simulink library "powerlib_modelsV2"  (Simulink 6.0)
settings: Solver=ode45  SolverMode=SingleTasking  StartTime=0.0  StopTime=10.0  RelTol=1e-3
values from neighbouring files (symbols this model uses):
  Ts = get(handles.edit1,'string')    [powergui.m]
undefined symbols (not defined in the file or in its folder): A, Ac, B, Bc, C, Cc, Cs, Current, damp, Dc, Dd, DiscIntNeverNeededParam, dref, dwo, exc, F, fb, gate, GH, GHd, GI, GId, GL, GLd, H, HT, hyd, ib, ib2, io, isfinite, j, K, Kd, Kg, L, Lad, Laq, lim, LIM, Ll, Llfd, Llkd, Llkq1, Llkq2, Llr, Lls, LowerFlux, N, N2, Nb, Nb2, nb_arm, p, Par_HarmoA_pu, Par_HarmoB_pu, Par_Timing_Harmo, Par_Timing_Variation, Par_Vps, Pb ... (+57)
libraries: powerlib_extras x14
(part 7 of 11)

== system powerlib_modelsV2/Continuous/simplified_sync_mach/Subsystem ==
  i : Inport  Port=1  LatchInput=off
  v : Inport  Port=2  LatchInput=off
  e : Inport  Port=3  LatchInput=off
  theta : Inport  Port=4  LatchInput=off
  wm : Inport  Port=5  LatchInput=off
  Pe : Inport  Port=6  LatchInput=off
  Gain : Gain  Gain=[ ib2*ones(3,1); Vb3*ones(6,1); 1; Nb; Pb ]  SaturateOnIntegerOverflow=on
  Mux : Mux  Inputs=[ 3 3 3 1 1 1 ]
  * : Outport  InitialOutput=0
  wires:
  Gain/1 -> */1
  Mux/1 -> Gain/1
  Pe/1 -> Mux/6
  wm/1 -> Mux/5
  theta/1 -> Mux/4
  e/1 -> Mux/3
  v/1 -> Mux/2
  i/1 -> Mux/1

== system powerlib_modelsV2/Continuous/simplified_sync_mach/Vt ==
  note: This subsystem either converts 2 line-to-line voltages to 3 line-to-neutral voltages (internal neutral)
      | and computes floating neutral voltage or directly passes Van,Vbn,Vcn if 4-wire connection.
  V : Inport  Port=1  LatchInput=off
  1_Vb : Gain  Gain=1/Vb  SaturateOnIntegerOverflow=on
  Constant : Constant  Orientation=left  Value=v6==1
  Constant1 : Constant  Value=0
  Constant2 : Constant  Value=0
  Data Type  Conversion1 : DataTypeConversion  Orientation=left  SaturateOnIntegerOverflow=on  RndMeth=Zero
  Data Type  Conversion2 : DataTypeConversion  SaturateOnIntegerOverflow=on  RndMeth=Zero
  Fcn : Fcn  Expr=u[1]
  Fcn1 : Fcn  Expr=u[2]
  Fcn2 : Fcn  Expr=u[3]
  Gain : Gain  Gain=1/3  SaturateOnIntegerOverflow=on
  LL2LN : Subsystem  TreatAsAtomicUnit=on
  Logical Operator : Logic  Operator=NOT
  Mux : Mux  Inputs=2
  Mux1 : Mux  Inputs=3
  Product : Product  SaturateOnIntegerOverflow=on  InputSameDT=on
  Sum : Sum  Inputs=+  SaturateOnIntegerOverflow=on  InputSameDT=on
  Sum1 : Sum  Inputs=|++  SaturateOnIntegerOverflow=on  InputSameDT=on
  Switch2 : Switch  Threshold=0.5  InputSameDT=on
  Vn : Outport  InitialOutput=0
  Vabc : Outport  Port=2  InitialOutput=0
  wires:
  Data Type  Conversion2/1 -> Product/1
  Logical Operator/1 -> Data Type  Conversion2/1
  Data Type  Conversion1/1 -> Logical Operator/1
  Constant/1 -> Data Type  Conversion1/1, LL2LN/Enable, Switch2/2
  Sum/1 -> Gain/1
  Gain/1 -> Switch2/1
  Constant2/1 -> Switch2/3
  Switch2/1 -> Vn/1
  LL2LN/1(Out1) -> Sum/1, Sum1/1
  Sum1/1 -> Vabc/1
  Constant1/1 -> Mux/2
  Mux/1 -> Fcn/1, Fcn1/1, Fcn2/1
  Fcn/1 -> Mux1/1
  Fcn1/1 -> Mux1/2
  Fcn2/1 -> Mux1/3
  Mux1/1 -> Product/2
  Product/1 -> Sum1/2
  V/1 -> 1_Vb/1
  1_Vb/1 -> LL2LN/1(In1), Mux/1

== system powerlib_modelsV2/Continuous/simplified_sync_mach/Z ==
  note: This subsystem models the internal impedance of
      | the machine, which consists of  a series RL circuit.
  e : Inport  Port=1  LatchInput=off
  v : Inport  Port=2  LatchInput=off
  1/L : Gain  Gain=web_psb/L  SaturateOnIntegerOverflow=on
  Integrator3 : Integrator  InitialCondition=io
  R : Gain  Orientation=left  Gain=R  SaturateOnIntegerOverflow=on
  Sum5 : Sum  Inputs=-+-  SaturateOnIntegerOverflow=on  InputSameDT=on
  i : Outport  InitialOutput=0
  wires:
  Integrator3/1 -> i/1, R/1
  1/L/1 -> Integrator3/1
  v/1 -> Sum5/3
  Sum5/1 -> 1/L/1
  R/1 -> Sum5/1
  e/1 -> Sum5/2

== system powerlib_modelsV2/Continuous/simplified_sync_mach/gen ==
  note: This subsystem generates the 3 line-to-neutral voltages inside the machine.
  theta : Inport  Port=1  LatchInput=off
  E : Inport  Port=2  LatchInput=off
  Vn : Inport  Port=3  LatchInput=off
  1_Vb2 : Gain  Gain=1/Vb2  SaturateOnIntegerOverflow=on
  Mux : Mux  Inputs=3
  Product : Product  SaturateOnIntegerOverflow=on  InputSameDT=on
  Sum : Sum  Inputs=|++  SaturateOnIntegerOverflow=on  InputSameDT=on
  Sum1 : Sum  Orientation=down  Inputs=--  SaturateOnIntegerOverflow=on  InputSameDT=on
  rem(wt,2pi) : Fcn  Expr=rem(u[1],2*pi)
  sin(a) : Fcn  Expr=sin(u)
  sin(b) : Fcn  Expr=sin(u-pi23)
  e : Outport  InitialOutput=0
  wires:
  rem(wt,2pi)/1 -> sin(a)/1, sin(b)/1
  theta/1 -> rem(wt,2pi)/1
  sin(a)/1 -> Sum1/2, Mux/1
  Sum1/1 -> Mux/3
  sin(b)/1 -> Sum1/1, Mux/2
  E/1 -> 1_Vb2/1
  1_Vb2/1 -> Product/2
  Vn/1 -> Sum/2
  Mux/1 -> Product/1
  Product/1 -> Sum/1
  Sum/1 -> e/1

== system powerlib_modelsV2/Continuous/simplified_sync_mach/mechanics ==
  Pm : Inport  Port=1  LatchInput=off
  Pe : Inport  Port=2  LatchInput=off
  1_(2*H) : Gain  Gain=1/(2*H)  SaturateOnIntegerOverflow=on
  1_Pb : Gain  Gain=1/Pb  SaturateOnIntegerOverflow=on
  Gain : Gain  Orientation=left  Gain=Kd  SaturateOnIntegerOverflow=on
  Integrator : Integrator  InitialCondition=dwo
  Integrator1 : Integrator  InitialCondition=tho
  Mux1 : Mux  Inputs=2
  Sum : Sum  SaturateOnIntegerOverflow=on  InputSameDT=on
  Sum1 : Sum  Inputs=+-  SaturateOnIntegerOverflow=on  InputSameDT=on
  Sum2 : Sum  Inputs=-+  SaturateOnIntegerOverflow=on  InputSameDT=on
  div : Fcn  Expr=u[2]/u[1]
      mask Display: disp('division')
  nom. speed : Constant
  web_psb : Gain  Gain=web_psb  SaturateOnIntegerOverflow=on
  theta_e : Outport  InitialOutput=0
  wm : Outport  Port=2  InitialOutput=0
  wires:
  Pm/1 -> 1_Pb/1
  1_Pb/1 -> Sum2/2
  web_psb/1 -> Integrator1/1
  Integrator1/1 -> theta_e/1
  Mux1/1 -> div/1
  Pe/1 -> Sum2/1
  Sum2/1 -> Mux1/2
  Sum/1 -> Mux1/1, wm/1, web_psb/1
  1_(2*H)/1 -> Integrator/1
  div/1 -> Sum1/1
  Gain/1 -> Sum1/2
  Sum1/1 -> 1_(2*H)/1
  Integrator/1 -> Sum/2, Gain/1
  nom. speed/1 -> Sum/1

== system powerlib_modelsV2/Continuous/simplified_sync_mach/wattmeter ==
  note: This subsystem computes the total electrical
      | power delivered or absorbed by the machine.
  i : Inport  Port=1  LatchInput=off
  v : Inport  Port=2  LatchInput=off
  2_3 : Gain  Gain=2/3  SaturateOnIntegerOverflow=on
  Product : Product  SaturateOnIntegerOverflow=on  InputSameDT=on
  Sum : Sum  Inputs=+  SaturateOnIntegerOverflow=on  InputSameDT=on
  Pe : Outport  InitialOutput=0
  wires:
  Product/1 -> Sum/1
  i/1 -> Product/1
  v/1 -> Product/2
  Sum/1 -> 2_3/1
  2_3/1 -> Pe/1

== system powerlib_modelsV2/Continuous/synchronous_machine/Delta angle ==
  Vq : Inport  Port=1  PortDimensions=1  LatchInput=off
  Vd : Inport  Port=2  PortDimensions=1  LatchInput=off
  Cartesian to Polar : Subsystem
      mask Type: Cart2Polar
      mask Description:
      | Transformation from cartesian to polar coordinates.
      | [x, y] -> [r, theta]
      | 
      | r = sqrt(x^2 + y^2);
      | theta = atan(y/x);
      mask Help: Unmask this block for more help.
      mask Display: plot(0,0,100,100,[24,20,15,20,20],[85,95,85,95,20],[80,20,95,85,95,85],[70,20,20,15,20,24],[56,56,55,52,50,46],[20,26,31,35,38,42])
  Radians to Degrees : Subsystem
      mask Type: RadiansToDegrees
      mask Description:
      | Conversion from Radians to Degrees.
      | 
      | D=180/pi*R
      mask Help: This block converts from Radians to Degrees.
      mask Display: disp('R2D')
  Terminator2 : Terminator
  delta : Outport
  wires:
  Cartesian to Polar/2(theta) -> Radians to Degrees/1(Radians in)
  Cartesian to Polar/1(r) -> Terminator2/1
  Vq/1 -> Cartesian to Polar/1(x)
  Radians to Degrees/1(Degrees out) -> delta/1  "delta"
  Vd/1 -> Cartesian to Polar/2(y)

== system powerlib_modelsV2/Continuous/synchronous_machine/PQ ==
  note: PQ Measurement:
  note: Q = Vq*Id-Vd*Iq
  note: P = Vd*Id + Vq*Iq
  Vq : Inport  Port=1  PortDimensions=1  LatchInput=off
  Vd : Inport  Port=2  PortDimensions=1  LatchInput=off
  Iq : Inport  Port=3  PortDimensions=2  LatchInput=off
  Demux1 : Demux  Outputs=[1,1]
  Gain : Gain  Gain=Gain1  SaturateOnIntegerOverflow=on
  Gain1 : Gain  Gain=Gain1  SaturateOnIntegerOverflow=on
  Product{2..5} (4 alike) : Product  SaturateOnIntegerOverflow=on  InputSameDT=on
  Sum : Sum  SaturateOnIntegerOverflow=on  InputSameDT=on
  Sum1 : Sum  Inputs=+-  SaturateOnIntegerOverflow=on  InputSameDT=on
  Peo : Outport
  Qeo : Outport  Port=2
  wires:
  Demux1/2 -> Product4/2, Product3/2
  Vq/1 -> Product4/1, Product2/1
  Vd/1 -> Product5/1, Product3/1
  Sum1/1 -> Gain1/1  "Qeo"
  Sum/1 -> Gain/1  "Peo"
  Product5/1 -> Sum1/2
  Product4/1 -> Sum1/1
  Product3/1 -> Sum/2
  Product2/1 -> Sum/1
  Gain/1 -> Peo/1
  Gain1/1 -> Qeo/1
  Iq/1 -> Demux1/1
  Demux1/1 -> Product2/2, Product5/2

== system powerlib_modelsV2/Continuous/synchronous_machine/Subsystem ==
  Vf : Inport  Port=1  PortDimensions=1  LatchInput=off
  Constant : Constant  Value=excAxis
  Ground2 : Ground
  Switch : Switch  Threshold=1.5  InputSameDT=on
  Switch1 : Switch  Threshold=1.5  InputSameDT=on
  Vkq1 : Outport
  Vfd : Outport  Port=2
  wires:
  Ground2/1 -> Switch1/1, Switch/3
  Vf/1 -> Switch1/3, Switch/1
  Constant/1 -> Switch/2, Switch1/2
  Switch1/1 -> Vfd/1
  Switch/1 -> Vkq1/1

== system powerlib_modelsV2/Continuous/synchronous_machine/abc2qd ==
  note: This subsystem converts Vab and Vbc to Vd,Vq. The sine and cosine com-
      | puted here are sent to the inverse transformation subsystem qd/abc.
  v : Inport  Port=1  PortDimensions=2  LatchInput=off
  theta : Inport  Port=2  PortDimensions=1  LatchInput=off
  1_Vb : Gain  Gain=1/Vb  SaturateOnIntegerOverflow=on
  Elementary Math : ElementaryMath
  Elementary Math1 : ElementaryMath  Operator=cos
  Fcn2 : Fcn  Expr=(u[4]*(2*u[1]+u[2]) + (sqrt3*u[2]*u[3])) * one_third
  Fcn3 : Fcn  Expr=(u[3]*(2*u[1]+u[2]) + (-sqrt3*u[2]*u[4])) * one_third
  Mux1 : Mux  Inputs=[ 2 2 ]
  Mux3 : Mux  Inputs=2
  cos,sin : Outport  InitialOutput=0
  vq : Outport  Port=2  InitialOutput=0
  vd : Outport  Port=3  InitialOutput=0
  wires:
  1_Vb/1 -> Mux1/1
  v/1 -> 1_Vb/1
  Mux1/1 -> Fcn2/1, Fcn3/1
  Mux3/1 -> Mux1/2, cos,sin/1
  theta/1 -> Elementary Math/1, Elementary Math1/1
  Elementary Math/1 -> Mux3/1
  Elementary Math1/1 -> Mux3/2
  Fcn2/1 -> vq/1  "vq"
  Fcn3/1 -> vd/1  "vd"

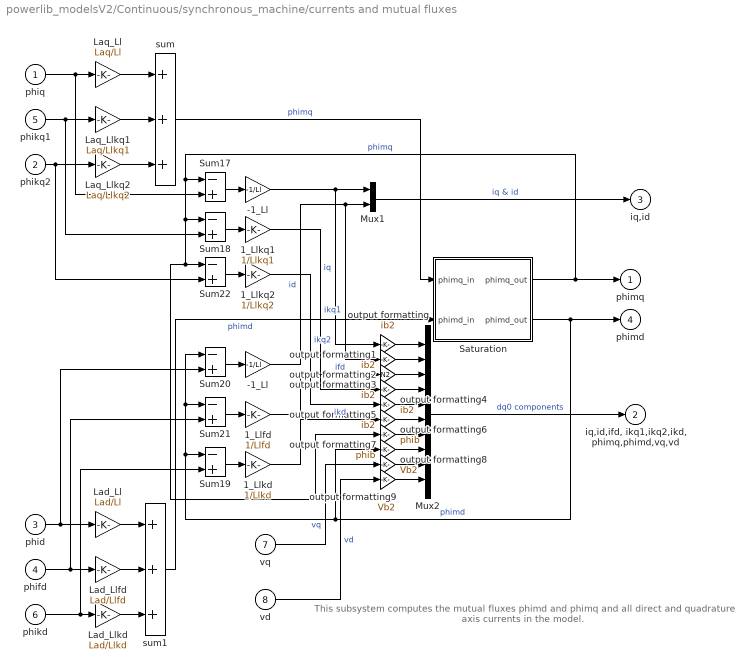
== system powerlib_modelsV2/Continuous/synchronous_machine/currents and mutual fluxes ==
  note: This subsystem computes the mutual fluxes phimd
      | and phimq and all direct and quadrature axis
      | currents in the model.
  phiq : Inport  Port=1  PortDimensions=1  LatchInput=off
  phikq2 : Inport  Port=2  PortDimensions=1  LatchInput=off
  phid : Inport  Port=3  PortDimensions=1  LatchInput=off
  phifd : Inport  Port=4  PortDimensions=1  LatchInput=off
  phikq1 : Inport  Port=5  PortDimensions=1  LatchInput=off
  phikd : Inport  Port=6  PortDimensions=1  LatchInput=off
  vq : Inport  Port=7  PortDimensions=1  LatchInput=off
  vd : Inport  Port=8  PortDimensions=1  LatchInput=off
  -1_Ll : Gain  Gain=-1/Ll  SaturateOnIntegerOverflow=on
  "-1_Ll " : Gain  Gain=-1/Ll  SaturateOnIntegerOverflow=on
  1_Llfd : Gain  Gain=1/Llfd  SaturateOnIntegerOverflow=on
  1_Llkd : Gain  Gain=1/Llkd  SaturateOnIntegerOverflow=on
  1_Llkq1 : Gain  Gain=1/Llkq1  SaturateOnIntegerOverflow=on
  1_Llkq2 : Gain  Gain=1/Llkq2  SaturateOnIntegerOverflow=on
  Lad_Ll : Gain  Gain=Lad/Ll  SaturateOnIntegerOverflow=on
  Lad_Llfd : Gain  Gain=Lad/Llfd  SaturateOnIntegerOverflow=on
  Lad_Llkd : Gain  Gain=Lad/Llkd  SaturateOnIntegerOverflow=on
  Laq_Ll : Gain  Gain=Laq/Ll  SaturateOnIntegerOverflow=on
  Laq_Llkq1 : Gain  Gain=Laq/Llkq1  SaturateOnIntegerOverflow=on
  Laq_Llkq2 : Gain  Gain=Laq/Llkq2  SaturateOnIntegerOverflow=on
  Mux1 : Mux  Inputs=2
  Mux2 : Mux  Inputs=[1,1,1,1,1,1,1,1,1,1]
  Saturation : Subsystem
  Sum{17..22} (6 alike) : Sum  Inputs=-+  SaturateOnIntegerOverflow=on  InputSameDT=on
  output formatting{,1,3..5} (5 alike) : Gain  Gain=ib2  SaturateOnIntegerOverflow=on
  output formatting2 : Gain  Gain=N2  SaturateOnIntegerOverflow=on
  output formatting6 : Gain  Gain=phib  SaturateOnIntegerOverflow=on
  output formatting7 : Gain  Gain=phib  SaturateOnIntegerOverflow=on
  output formatting8 : Gain  Gain=Vb2  SaturateOnIntegerOverflow=on
  output formatting9 : Gain  Gain=Vb2  SaturateOnIntegerOverflow=on
  sum : Sum  Inputs=+++  SaturateOnIntegerOverflow=on  InputSameDT=on
  sum1 : Sum  Inputs=+++  SaturateOnIntegerOverflow=on  InputSameDT=on
  phimq : Outport  InitialOutput=0
  "iq,id,ifd, ikq1,ikq2,ikd, phimq,phimd,vq,vd" : Outport  Port=2  InitialOutput=0
  iq,id : Outport  Port=3  InitialOutput=0
  phimd : Outport  Port=4  InitialOutput=0
  wires:
  Saturation/2(phimd_out) -> Sum19/1, Sum21/1, Sum20/1, output formatting7/1, phimd/1  "phimd"
  Saturation/1(phimq_out) -> Sum17/1, Sum22/1, output formatting6/1, Sum18/1, phimq/1  "phimq"
  sum1/1 -> Saturation/2(phimd_in)  "phimd"
  sum/1 -> Saturation/1(phimq_in)  "phimq"
  1_Llkq2/1 -> output formatting4/1  "ikq2"
  1_Llkq1/1 -> output formatting3/1  "ikq1"
  Sum20/1 -> "-1_Ll "/1
  "-1_Ll "/1 -> Mux1/2, output formatting1/1  "id"
  Sum21/1 -> 1_Llfd/1
  Sum19/1 -> 1_Llkd/1
  1_Llfd/1 -> output formatting2/1  "ifd"
  1_Llkd/1 -> output formatting5/1  "ikd"
  Sum18/1 -> 1_Llkq1/1
  Sum17/1 -> -1_Ll/1
  Sum22/1 -> 1_Llkq2/1
  -1_Ll/1 -> Mux1/1, output formatting/1  "iq"
  Mux1/1 -> iq,id/1  "iq & id"
  Lad_Llkd/1 -> sum1/3
  Lad_Llfd/1 -> sum1/2
  Lad_Ll/1 -> sum1/1
  phifd/1 -> Lad_Llfd/1, Sum21/2
  phid/1 -> Sum20/2, Lad_Ll/1
  phikd/1 -> Lad_Llkd/1, Sum19/2
  phiq/1 -> Laq_Ll/1, Sum17/2
  Laq_Ll/1 -> sum/1
  Laq_Llkq2/1 -> sum/3
  Laq_Llkq1/1 -> sum/2
  phikq2/1 -> Laq_Llkq2/1, Sum22/2
  phikq1/1 -> Laq_Llkq1/1, Sum18/2
  vq/1 -> output formatting8/1  "vq"
  vd/1 -> output formatting9/1  "vd"
  Mux2/1 -> "iq,id,ifd, ikq1,ikq2,ikd, phimq,phimd,vq,vd"/1  "dq0 components"
  output formatting/1 -> Mux2/1
  output formatting1/1 -> Mux2/2
  output formatting2/1 -> Mux2/3
  output formatting3/1 -> Mux2/4
  output formatting4/1 -> Mux2/5
  output formatting5/1 -> Mux2/6
  output formatting6/1 -> Mux2/7
  output formatting7/1 -> Mux2/8
  output formatting8/1 -> Mux2/9
  output formatting9/1 -> Mux2/10

== system powerlib_modelsV2/Continuous/synchronous_machine/mec ==
  note: This subsystem models the mechanical part of the machine.
  note: Attention: Te tjrs en p.u
  "iq,id " : Inport  Port=1  PortDimensions=2  LatchInput=off
  phid : Inport  Port=2  PortDimensions=1  LatchInput=off
  phiq : Inport  Port=3  PortDimensions=1  LatchInput=off
  Pm : Inport  Port=4  PortDimensions=1  LatchInput=off
  1_(2H) : Gain  Gain=1/(2*H)  SaturateOnIntegerOverflow=on
  1_Pb : Gain  Gain=1/Pb  SaturateOnIntegerOverflow=on
  Clock : Clock
      settings: Decimation=10
  F : Gain  Orientation=left  Gain=F  SaturateOnIntegerOverflow=on
  Fcn1 : Fcn  Expr=rem(u,2*pi)
  Integrator : Integrator  InitialCondition=dwo
  Integrator1 : Integrator  InitialCondition=tho
  Integrator2 : Integrator  InitialCondition=tho
  Mux : Mux  Inputs=[ 1 1 2 ]
  Mux1 : Mux  Inputs=2
  Mux2 : Mux  Inputs=[1,1,1,1,1,1]
  Product : Product  SaturateOnIntegerOverflow=on  InputSameDT=on
  Sum : Sum  SaturateOnIntegerOverflow=on  InputSameDT=on
  Sum2 : Sum  Inputs=+--  SaturateOnIntegerOverflow=on  InputSameDT=on
  Sum3 : Sum  SaturateOnIntegerOverflow=on  InputSameDT=on
  Te : Fcn  Expr=u[1]*u[3]-u[2]*u[4]
  div : Fcn  Expr=u[2]/u[1]
      mask Display: disp('/')
  nom. speed : Constant
  theta : Gain  Gain=180/pi  SaturateOnIntegerOverflow=on
  units : Gain  Gain=Nb  SaturateOnIntegerOverflow=on
  units1 : Gain  Gain=Pb  SaturateOnIntegerOverflow=on
  units2 : Gain  Gain=Pb/Nb  SaturateOnIntegerOverflow=on
  web1 : Gain  Gain=web_psb  SaturateOnIntegerOverflow=on
  web2 : Gain  Gain=web_psb  SaturateOnIntegerOverflow=on
  web3 : Gain  Gain=web_psb  SaturateOnIntegerOverflow=on
  misc : Outport  InitialOutput=0
  thetae : Outport  Port=2  InitialOutput=0
  we : Outport  Port=3  InitialOutput=0
  wires:
  Integrator2/1 -> Sum3/1, Mux2/1  "d_theta (rad)"
  web2/1 -> Sum3/2
  Clock/1 -> web2/1
  web1/1 -> Integrator2/1
  Integrator/1 -> web1/1, F/1, Mux2/4, Sum/2  "dw"
  Product/1 -> units1/1  "Pe"
  nom. speed/1 -> Sum/1
  1_(2H)/1 -> Integrator/1
  div/1 -> Sum2/1
  phiq/1 -> Mux/2
  phid/1 -> Mux/1
  "iq,id "/1 -> Mux/3
  Te/1 -> Sum2/2, Product/2, units2/1  "Te"
  Mux/1 -> Te/1
  Mux1/1 -> div/1
  Pm/1 -> 1_Pb/1
  1_Pb/1 -> Mux1/2
  F/1 -> Sum2/3
  Sum2/1 -> 1_(2H)/1
  Sum/1 -> Product/1, web3/1, units/1, we/1, Mux1/1  "n"
  Sum3/1 -> thetae/1
  web3/1 -> Integrator1/1
  Integrator1/1 -> Fcn1/1  "d_theta (rad)"
  Fcn1/1 -> theta/1
  theta/1 -> Mux2/5  "theta"
  Mux2/1 -> misc/1  "Mechanical"
  units/1 -> Mux2/2  "n"
  units1/1 -> Mux2/3  "Pe"
  units2/1 -> Mux2/6  "Te"

== system powerlib_modelsV2/Continuous/synchronous_machine/phid ==
  note: This subsystem computes the direct axis flux phid.
  w : Inport  Port=1  PortDimensions=1  LatchInput=off
  phiq : Inport  Port=2  PortDimensions=1  LatchInput=off
  vd : Inport  Port=3  PortDimensions=1  LatchInput=off
  phimd : Inport  Port=4  PortDimensions=1  LatchInput=off
  Product1 : Product  SaturateOnIntegerOverflow=on  InputSameDT=on
  Rs_Ll : Gain  Gain=Rs/Ll  SaturateOnIntegerOverflow=on
  Sum2 : Sum  Inputs=+++  SaturateOnIntegerOverflow=on  InputSameDT=on
  Sum9 : Sum  Inputs=+-  SaturateOnIntegerOverflow=on  InputSameDT=on
  int : Integrator  InitialCondition=phido
  web_psb : Gain  Gain=web_psb  SaturateOnIntegerOverflow=on
  phid : Outport  InitialOutput=0
  wires:
  phimd/1 -> Sum9/1
  vd/1 -> Sum2/2
  phiq/1 -> Product1/2
  w/1 -> Product1/1
  Product1/1 -> Sum2/1
  Sum9/1 -> Rs_Ll/1
  Rs_Ll/1 -> Sum2/3
  Sum2/1 -> web_psb/1
  web_psb/1 -> int/1
  int/1 -> phid/1, Sum9/2

== system powerlib_modelsV2/Continuous/synchronous_machine/phifd ==
  note: This subsystem computes the field flux phifd.
  vfd : Inport  Port=1  PortDimensions=1  LatchInput=off
  phimd : Inport  Port=2  PortDimensions=1  LatchInput=off
  N : Gain  Gain=N  SaturateOnIntegerOverflow=on
  Rf_Llfd : Gain  Gain=Rf/Llfd  SaturateOnIntegerOverflow=on
  Sum10 : Sum  Inputs=+-  SaturateOnIntegerOverflow=on  InputSameDT=on
  Sum3 : Sum  SaturateOnIntegerOverflow=on  InputSameDT=on
  int : Integrator  InitialCondition=phifdo
  web_psb : Gain  Gain=web_psb  SaturateOnIntegerOverflow=on
  phifd : Outport  InitialOutput=0
  wires:
  N/1 -> Sum3/1
  vfd/1 -> N/1
  Rf_Llfd/1 -> Sum3/2
  Sum10/1 -> Rf_Llfd/1
  phimd/1 -> Sum10/1
  web_psb/1 -> int/1
  int/1 -> phifd/1, Sum10/2
  Sum3/1 -> web_psb/1

== system powerlib_modelsV2/Continuous/synchronous_machine/phikd ==
  note: This subsystem computes the direct axis damper flux phikd.
  phimd : Inport  Port=1  PortDimensions=1  LatchInput=off
  vkd : Inport  Port=2  PortDimensions=1  LatchInput=off
  Rkd_Llkd : Gain  Gain=Rkd/Llkd  SaturateOnIntegerOverflow=on
  Sum11 : Sum  Inputs=-+  SaturateOnIntegerOverflow=on  InputSameDT=on
  Sum4 : Sum  SaturateOnIntegerOverflow=on  InputSameDT=on
  int : Integrator  InitialCondition=phikdo
  web_psb : Gain  Gain=web_psb  SaturateOnIntegerOverflow=on
  phikd : Outport  InitialOutput=0
  wires:
  Rkd_Llkd/1 -> Sum4/1
  Sum11/1 -> Rkd_Llkd/1
  phimd/1 -> Sum11/2
  vkd/1 -> Sum4/2
  web_psb/1 -> int/1
  int/1 -> phikd/1, Sum11/1
  Sum4/1 -> web_psb/1

== system powerlib_modelsV2/Continuous/synchronous_machine/phikq1 ==
  note: This subsystem computes the quadrature axis damper flux phikq.
  phimq : Inport  Port=1  PortDimensions=1  LatchInput=off
  vkq1 : Inport  Port=2  PortDimensions=1  LatchInput=off
  Rkq1_Llkq1 : Gain  Gain=Rkq1/Llkq1  SaturateOnIntegerOverflow=on
  Sum1 : Sum  SaturateOnIntegerOverflow=on  InputSameDT=on
  Sum7 : Sum  Inputs=-+  SaturateOnIntegerOverflow=on  InputSameDT=on
  int : Integrator  InitialCondition=phikq1o
  web_psb : Gain  Gain=web_psb  SaturateOnIntegerOverflow=on
  phikq1 : Outport  InitialOutput=0
  wires:
  int/1 -> Sum7/1, phikq1/1
  web_psb/1 -> int/1
  vkq1/1 -> Sum1/2
  phimq/1 -> Sum7/2
  Sum1/1 -> web_psb/1
  Sum7/1 -> Rkq1_Llkq1/1
  Rkq1_Llkq1/1 -> Sum1/1

== system powerlib_modelsV2/Continuous/synchronous_machine/phikq2 ==
  note: This subsystem computes the quadrature axis damper flux phikq2.
  vkq2 : Inport  Port=1  PortDimensions=1  LatchInput=off
  phimq : Inport  Port=2  PortDimensions=1  LatchInput=off
  Enabled integrator : Subsystem  TreatAsAtomicUnit=on
      mask Display: disp('1/s')
  Rkq2_Llkq2 : Gain  Gain=Rkq2/Llkq2  SaturateOnIntegerOverflow=on
  Sum1 : Sum  SaturateOnIntegerOverflow=on  InputSameDT=on
  Sum7 : Sum  Inputs=-+  SaturateOnIntegerOverflow=on  InputSameDT=on
  web_psb : Gain  Gain=web_psb  SaturateOnIntegerOverflow=on
  wref : Constant  Value=isfinite(Llkq2)
  phikq2 : Outport  InitialOutput=0
  wires:
  wref/1 -> Enabled integrator/Enable
  Enabled integrator/1(Out1) -> phikq2/1, Sum7/1
  web_psb/1 -> Enabled integrator/1(In1)
  Sum7/1 -> Rkq2_Llkq2/1
  vkq2/1 -> Sum1/2
  Rkq2_Llkq2/1 -> Sum1/1
  Sum1/1 -> web_psb/1
  phimq/1 -> Sum7/2

== system powerlib_modelsV2/Continuous/synchronous_machine/phiq ==
  note: This subsystem computes the quadrature axis flux phiq.
  vq : Inport  Port=1  PortDimensions=1  LatchInput=off
  w : Inport  Port=2  PortDimensions=1  LatchInput=off
  phid : Inport  Port=3  PortDimensions=1  LatchInput=off
  phimq : Inport  Port=4  PortDimensions=1  LatchInput=off
  Product2 : Product  SaturateOnIntegerOverflow=on  InputSameDT=on
  Rs_Ll : Gain  Gain=Rs/Ll  SaturateOnIntegerOverflow=on
  Sum : Sum  Inputs=+-+  SaturateOnIntegerOverflow=on  InputSameDT=on
  Sum6 : Sum  Inputs=+-  SaturateOnIntegerOverflow=on  InputSameDT=on
  int1 : Integrator  InitialCondition=phiqo
  web_psb : Gain  Gain=web_psb  SaturateOnIntegerOverflow=on
  phiq : Outport  InitialOutput=0
  wires:
  Sum/1 -> web_psb/1
  Rs_Ll/1 -> Sum/3
  Sum6/1 -> Rs_Ll/1
  Product2/1 -> Sum/2
  vq/1 -> Sum/1
  w/1 -> Product2/1
  phid/1 -> Product2/2
  phimq/1 -> Sum6/1
  web_psb/1 -> int1/1
  int1/1 -> phiq/1, Sum6/2

== system powerlib_modelsV2/Continuous/synchronous_machine/qd2abc ==
  note: This subsystem converts id,iq to ia,ib,ic.
  sin,cos : Inport  Port=1  PortDimensions=2  LatchInput=off
  iq,id : Inport  Port=2  PortDimensions=2  LatchInput=off
  Fcn : Fcn  Expr=u[3]*u[2] + u[4]*u[1]
  Fcn1 : Fcn  Expr=(u[2]*(-u[3]-sqrt3*u[4]) + u[1]*(sqrt3*u[3]-u[4]))*0.5
  Mux : Mux  Inputs=[ 2 2 ]
  Mux1 : Mux  Inputs=[1,1,1]
  Mux1_ : Mux  Inputs=3
  Sum : Sum  Orientation=down  Inputs=--  SaturateOnIntegerOverflow=on  InputSameDT=on
  ib : Gain  Gain=ib  SaturateOnIntegerOverflow=on
  output formatting : Gain  Gain=ib2  SaturateOnIntegerOverflow=on
  output formatting1 : Gain  Gain=ib2  SaturateOnIntegerOverflow=on
  output formatting2 : Gain  Gain=ib2  SaturateOnIntegerOverflow=on
  is(A) : Outport  InitialOutput=0
  is(pu) : Outport  Port=2  InitialOutput=0
  wires:
  iq,id/1 -> Mux/2
  sin,cos/1 -> Mux/1
  Mux/1 -> Fcn1/1, Fcn/1
  Mux1_/1 -> ib/1
  Sum/1 -> Mux1_/3, output formatting2/1  "is_c"
  Fcn/1 -> Sum/1, Mux1_/1, output formatting/1  "is_a"
  Fcn1/1 -> Sum/2, Mux1_/2, output formatting1/1  "is_b"
  ib/1 -> is(A)/1
  Mux1/1 -> is(pu)/1  "Stator currents"
  output formatting/1 -> Mux1/1  "is_a"
  output formatting1/1 -> Mux1/2  "is_b"
  output formatting2/1 -> Mux1/3  "is_c"

== system powerlib_modelsV2/Continuous/thyristor (logical)/Break Alg. Loop ==
  In1 : Inport  Port=1  LatchInput=off
  0 2 : Constant  Value=0.001
  Data Type  Conversion : DataTypeConversion  SaturateOnIntegerOverflow=on  RndMeth=Zero
  Data Type  Conversion1 : DataTypeConversion  SaturateOnIntegerOverflow=on  RndMeth=Zero
  Integrator : Integrator  LimitOutput=on  UpperSaturationLimit=0.00101
  R_device : Gain  Gain=1e7  SaturateOnIntegerOverflow=on
  Relational Operator1 : RelationalOperator  Operator=>  InputSameDT=on
  Vak-Vf-Ron*Iak : Sum  Inputs=+-  SaturateOnIntegerOverflow=on  InputSameDT=on
  Out1 : Outport
  wires:
  Relational Operator1/1 -> Data Type  Conversion/1
  0 2/1 -> Relational Operator1/2
  Integrator/1 -> Relational Operator1/1, Vak-Vf-Ron*Iak/2
  Vak-Vf-Ron*Iak/1 -> R_device/1
  R_device/1 -> Integrator/1
  Data Type  Conversion1/1 -> Vak-Vf-Ron*Iak/1
  In1/1 -> Data Type  Conversion1/1
  Data Type  Conversion/1 -> Out1/1

== system powerlib_modelsV2/Discrete/3_Phase_Prog_Source/Harmonic A generation ==
  Enable : Inport  Port=1  LatchInput=off
  Gain2 : Gain  Gain=2*pi*n_Harmo  SaturateOnIntegerOverflow=on
  Gain3 : Gain  Gain=pi/180  SaturateOnIntegerOverflow=on
  Multiport Switch : MultiPortSwitch  Inputs=3  InputSameDT=on
  Negative-sequence : Constant  Value=[0 2*pi/3 -2*pi/3]
  Phase_Harmo : Constant  Value=Phase_Harmo
  Phase_Harmo1 : Constant  Value=Mag_Harmo
  Phase_Harmo2 : Constant  Value=Seq_Harmo
  Positive-sequence : Constant  Value=[0 -2*pi/3 2*pi/3]
  Product : Product  SaturateOnIntegerOverflow=on  InputSameDT=on
  Product1 : Product  Inputs=3  SaturateOnIntegerOverflow=on  InputSameDT=on
  Sum : Sum  Inputs=+++  SaturateOnIntegerOverflow=on  InputSameDT=on
  Sum1 : Sum  SaturateOnIntegerOverflow=on  InputSameDT=on
  Trigonometric Function1 : Trigonometry
  Zero-sequence : Constant  Value=[0 0 0]
  t : DigitalClock  SampleTime=Ts
  valp_nom1 : Constant  Value=Freq_Vps
  valp_nom2 : Constant
  HarmoA : Outport
  wires:
  Gain3/1 -> Sum/2
  Phase_Harmo/1 -> Gain3/1
  Enable/1 -> Product1/1
  valp_nom2/1 -> Sum1/2
  Phase_Harmo2/1 -> Sum1/1
  Sum1/1 -> Multiport Switch/1
  Phase_Harmo1/1 -> Product1/2
  Product1/1 -> HarmoA/1
  Trigonometric Function1/1 -> Product1/3
  Product/1 -> Sum/1
  t/1 -> Product/1
  Gain2/1 -> Product/2
  valp_nom1/1 -> Gain2/1
  Negative-sequence/1 -> Multiport Switch/4
  Positive-sequence/1 -> Multiport Switch/3
  Zero-sequence/1 -> Multiport Switch/2
  Multiport Switch/1 -> Sum/3
  Sum/1 -> Trigonometric Function1/1

== system powerlib_modelsV2/Discrete/3_Phase_Prog_Source/Harmonic B generation ==
  Enable : Inport  Port=1  LatchInput=off
  Gain2 : Gain  Gain=2*pi*n_Harmo  SaturateOnIntegerOverflow=on
  Gain3 : Gain  Gain=pi/180  SaturateOnIntegerOverflow=on
  Multiport Switch : MultiPortSwitch  Inputs=3  InputSameDT=on
  Negative-sequence : Constant  Value=[0 2*pi/3 -2*pi/3]
  Phase_Harmo : Constant  Value=Phase_Harmo
  Phase_Harmo1 : Constant  Value=Mag_Harmo
  Phase_Harmo2 : Constant  Value=Seq_Harmo
  Positive-sequence : Constant  Value=[0 -2*pi/3 2*pi/3]
  Product : Product  SaturateOnIntegerOverflow=on  InputSameDT=on
  Product1 : Product  Inputs=3  SaturateOnIntegerOverflow=on  InputSameDT=on
  Sum : Sum  Inputs=+++  SaturateOnIntegerOverflow=on  InputSameDT=on
  Sum1 : Sum  SaturateOnIntegerOverflow=on  InputSameDT=on
  Trigonometric Function1 : Trigonometry
  Zero-sequence : Constant  Value=[0 0 0]
  t : DigitalClock  SampleTime=Ts
  valp_nom1 : Constant  Value=Freq_Vps
  valp_nom2 : Constant
  HarmoB : Outport
  wires:
  Gain3/1 -> Sum/2
  Phase_Harmo/1 -> Gain3/1
  Sum/1 -> Trigonometric Function1/1
  Multiport Switch/1 -> Sum/3
  Zero-sequence/1 -> Multiport Switch/2
  Positive-sequence/1 -> Multiport Switch/3
  Negative-sequence/1 -> Multiport Switch/4
  valp_nom1/1 -> Gain2/1
  Gain2/1 -> Product/2
  t/1 -> Product/1
  Product/1 -> Sum/1
  Trigonometric Function1/1 -> Product1/3
  Product1/1 -> HarmoB/1
  Phase_Harmo1/1 -> Product1/2
  Sum1/1 -> Multiport Switch/1
  Phase_Harmo2/1 -> Sum1/1
  valp_nom2/1 -> Sum1/2
  Enable/1 -> Product1/1

== system powerlib_modelsV2/Discrete/3_Phase_Prog_Source/Timer ==
  Clock : Clock
  Look-Up Table : Lookup  DialogController=Simulink.DDGSource  InputValues=tv  OutputValues=opv  SaturateOnIntegerOverflow=on
  Out : Outport
  wires:
  Look-Up Table/1 -> Out/1
  Clock/1 -> Look-Up Table/1

== system powerlib_modelsV2/Discrete/3_Phase_Prog_Source/Variation SubSystem ==
  VariationType : Inport  Port=1  LatchInput=off
  Constant : Constant  Value=2
  Constant1 : Constant  Value=0
  Constant2 : Constant
  Constant3 : Constant
  Constant4 : Constant  Value=0
  Constant5 : Constant  Value=0
  Data Type  Conversion1 : DataTypeConversion  SaturateOnIntegerOverflow=on  RndMeth=Zero
  Data Type  Conversion2 : DataTypeConversion  Orientation=up  SaturateOnIntegerOverflow=on  RndMeth=Zero
  Discrete-Time Integrator1 : DiscreteIntegrator  SampleTime=Ts  SaturateOnIntegerOverflow=on  ICPrevOutput=DiscIntNeverNeededParam  ICPrevScaledInput=DiscIntNeverNeededParam
  Gain1 : Gain  Gain=2*pi  SaturateOnIntegerOverflow=on
  Logical Operator : Logic
  Logical Operator1 : Logic  Orientation=up  Operator=NOT
  Multiport Switch1 : MultiPortSwitch  InputSameDT=on
  Product : Product  SaturateOnIntegerOverflow=on  InputSameDT=on
  Product1 : Product  SaturateOnIntegerOverflow=on  InputSameDT=on
  Product2 : Product  SaturateOnIntegerOverflow=on  InputSameDT=on
  Relational Operator : RelationalOperator  Operator===  InputSameDT=on
  Relational Operator1 : RelationalOperator  Operator===  InputSameDT=on
  Step : Step  Time=Ton_Variation  SampleTime=Ts
  Step1 : Step  Time=Toff_Variation  Before=1  After=0  SampleTime=Ts
  Switch{,1..3} (4 alike) : Switch  Threshold=0.5  InputSameDT=on
  Trigonometric Function1 : Trigonometry
  Unit Delay : UnitDelay  Orientation=left  SampleTime=Ts
  valp_nom6 : Constant  Value=VariationStep
  valp_nom7 : Constant  Value=VariationRate
  valp_nom8 : Constant  Value=VariationMag
  valp_nom9 : Constant  Value=VariationFreq
  Value : Outport
  wires:
  Data Type  Conversion1/1 -> Logical Operator/2
  Constant5/1 -> Multiport Switch1/5
  Logical Operator1/1 -> Logical Operator/1
  Logical Operator/1 -> Switch3/2
  Step1/1 -> Switch2/2, Data Type  Conversion2/1  "Toff"
  Constant3/1 -> Relational Operator1/2
  Switch3/1 -> Value/1
  Switch2/1 -> Switch3/3, Unit Delay/1
  Constant1/1 -> Switch3/1
  Unit Delay/1 -> Switch2/3
  Multiport Switch1/1 -> Switch2/1
  Step/1 -> Product2/2, Switch/2  "Ton"
  VariationType/1 -> Relational Operator/1, Relational Operator1/1, Multiport Switch1/1
  Discrete-Time Integrator1/1 -> Multiport Switch1/3, Product1/1  "Ramp"
  Product2/1 -> Multiport Switch1/2  "Step"
  valp_nom6/1 -> Product2/1
  Relational Operator/1 -> Switch1/2
  Switch/1 -> Discrete-Time Integrator1/1
  Constant/1 -> Relational Operator/2
  Switch1/1 -> Switch/1
  Constant4/1 -> Switch/3
  Constant2/1 -> Switch1/3
  valp_nom7/1 -> Switch1/1
  Product/1 -> Multiport Switch1/4  "Mod"
  Product1/1 -> Trigonometric Function1/1
  Gain1/1 -> Product1/2
  valp_nom9/1 -> Gain1/1
  valp_nom8/1 -> Product/1
  Trigonometric Function1/1 -> Product/2
  Data Type  Conversion2/1 -> Logical Operator1/1
  Relational Operator1/1 -> Data Type  Conversion1/1

== system powerlib_modelsV2/Discrete/Dynamic_Load/Discrete 3-phase PLL ==
  note: Pierre Giroux, Gilbert Sybille
      | Power System Laboratory, IREQ
      | Hydro-Quebec
  note: Discrete 3-phase PLL
  Vab_bc (pu) : Inport  Port=1  PortDimensions=2  LatchInput=off
  Constant4 : Constant  Value=2*pi
  Discrete PI Controller : powerlib_extras/Discrete  Control Blocks/Discrete PI Controller  Kp=Kp  Ki=Ki  Par_Limits=2*pi*Finit*[1.25 0.75]  Init=2*pi*Finit  Ts=Ts
  Discrete Rate Limiter : powerlib_extras/Discrete  Control Blocks/Discrete Rate Limiter  R=10  F=-10  Vinit=Finit  Ts=Ts
  Discrete Variable Frequency Mean value : powerlib_extras/Discrete Measurements/Discrete Variable Frequency Mean value  Finit=Finit  Fmin=45  Vinit=0  Ts=Ts
  Discrete  2nd-Order Filter : powerlib_extras/Discrete  Control Blocks/Discrete  2nd-Order Filter  FilterType=Lowpass  Fo=25  Zeta=0.707  Ts=Ts  Initialize=on  Vac_Init=[0 0 Finit]  Vdc_Init=Finit  PlotResponse=off  param1=[1 500 0.1]
  Discrete-Time Integrator : DiscreteIntegrator  InitialCondition=Phase_Init*pi/180  SampleTime=Ts  SaturateOnIntegerOverflow=on  ICPrevOutput=DiscIntNeverNeededParam  ICPrevScaledInput=DiscIntNeverNeededParam
  Gain10 : Gain  Gain=1/2/pi  SaturateOnIntegerOverflow=on
  Math Function : Math  Operator=mod  SaturateOnIntegerOverflow=on
  Mux2 : Mux  Inputs=2
  Trigonometric Function : Trigonometry
  Trigonometric Function2 : Trigonometry  Operator=cos
  Unit Delay : UnitDelay  X0=Finit  SampleTime=Ts
  abc_to_dq1 : Subsystem
  Freq : Outport
  Vd : Outport  Port=2
  Vq : Outport  Port=3
  sin_cos : Outport  Port=4
  wires:
  Discrete  2nd-Order Filter/1 -> Unit Delay/1
  Unit Delay/1 -> Discrete Variable Frequency Mean value/1, Freq/1
  Discrete Rate Limiter/1 -> Discrete  2nd-Order Filter/1
  Gain10/1 -> Discrete Rate Limiter/1
  Discrete PI Controller/1 -> Gain10/1, Discrete-Time Integrator/1  "W"
  Mux2/1 -> sin_cos/1, abc_to_dq1/2(sin_cos)
  Trigonometric Function2/1 -> Mux2/2
  Trigonometric Function/1 -> Mux2/1
  Math Function/1 -> Trigonometric Function2/1, Trigonometric Function/1
  Discrete-Time Integrator/1 -> Math Function/1
  Constant4/1 -> Math Function/2
  abc_to_dq1/2(vq) -> Discrete Variable Frequency Mean value/2, Vq/1  "Vq"
  Vab_bc (pu)/1 -> abc_to_dq1/1(Vab_bc)
  Discrete Variable Frequency Mean value/1 -> Discrete PI Controller/1
  abc_to_dq1/1(vd) -> Vd/1

== system powerlib_modelsV2/Discrete/Dynamic_Load/Positive Sequence  current ==
  note: kp=Vmin^(np-2)/Vo^np
      | kq=Vmin^(nq-2)/Vo^nq
  note: V<Vmin
      | Constant impedance load :
      |
      |  P=Po*kp*V^2
      | Q=Qo*kq*V^2
  note: V>Vmin :
      |
      |    P=Po*(V/Vo)^np
      |    Q=Qo*(V/Vo)^np
  note: I1= (S/V1)'
  V1(pu) : Inport  Port=1  PortDimensions=1  LatchInput=off
  S_ext : Inport  Port=2  PortDimensions=1  LatchInput=off
  Complex to Magnitude-Angle : ComplexToMagnitudeAngle  Output=Magnitude
  Complex to Real-Imag1 : ComplexToRealImag
  Conj1 : Math  Operator=conj  SaturateOnIntegerOverflow=on
  Math Function : Math  Operator=square  SaturateOnIntegerOverflow=on
  Mux1 : Mux  Inputs=3
  Mux2 : Mux  Inputs=2
  Mux3 : Mux  Inputs=2
  P0/ (Vo^np) : Gain  Gain=P0/(Mag_V0^np)  SaturateOnIntegerOverflow=on
  PQ_ext : Constant  Value=PQext
  Product : Product  Inputs=/*  SaturateOnIntegerOverflow=on  InputSameDT=on
  Q0/(Vo^nq) : Gain  Gain=Q0/(Mag_V0^nq)  SaturateOnIntegerOverflow=on
  Real-Imag to Complex : RealImagToComplex
  Switch1 : Switch  Threshold=0.5  InputSameDT=on
  Switch3 : Switch  Threshold=Vmin  InputSameDT=on
  Switch4 : Switch  Threshold=Vmin  InputSameDT=on
  TF_P : powerlib_extras/Discrete  Control Blocks/Discrete Lead-Lag  T1=Tp1  T2=Tp2  V_Init=P0  Ts=Ts
  TF_Q : powerlib_extras/Discrete  Control Blocks/Discrete Lead-Lag  T1=Tq1  T2=Tq2  V_Init=Q0  Ts=Ts
  V^nq : Fcn  Expr=u[1]^u[2]
  V^nq , : Fcn  Expr=u[1]^u[2]
  Vmin^(np-2) : Gain  Gain=Vmin^(np-2)  SaturateOnIntegerOverflow=on
  Vmin^(nq-2) : Gain  Gain=Vmin^(nq-2)  SaturateOnIntegerOverflow=on
  np : Constant  Value=np
  nq : Constant  Value=nq
  pu>V : Gain  Gain=Vnom*sqrt(3)/sqrt(2)  SaturateOnIntegerOverflow=on
  I1(A) : Outport
  VPQ : Outport  Port=2
  wires:
  Vmin^(nq-2)/1 -> Switch4/3
  V^nq ,/1 -> Switch3/1
  Vmin^(np-2)/1 -> Switch3/3
  Math Function/1 -> Vmin^(nq-2)/1, Vmin^(np-2)/1
  V^nq/1 -> Switch4/1
  V1(pu)/1 -> Complex to Magnitude-Angle/1, pu>V/1
  Mux3/1 -> V^nq/1
  nq/1 -> Mux3/2
  Mux2/1 -> V^nq ,/1
  np/1 -> Mux2/2
  Switch3/1 -> P0/ (Vo^np)/1
  Q0/(Vo^nq)/1 -> TF_Q/1
  P0/ (Vo^np)/1 -> TF_P/1
  Switch4/1 -> Q0/(Vo^nq)/1
  Product/1 -> Conj1/1
  Conj1/1 -> I1(A)/1
  Switch1/1 -> Product/2, Complex to Real-Imag1/1  "S=P+jQ"
  Real-Imag to Complex/1 -> Switch1/3  "S_dyn"
  S_ext/1 -> Switch1/1
  PQ_ext/1 -> Switch1/2
  pu>V/1 -> Product/1
  Complex to Magnitude-Angle/1 -> Math Function/1, Mux3/1, Mux2/1, Switch3/2, Switch4/2, Mux1/1
  Mux1/1 -> VPQ/1
  Complex to Real-Imag1/1 -> Mux1/2
  Complex to Real-Imag1/2 -> Mux1/3
  TF_P/1 -> Real-Imag to Complex/1
  TF_Q/1 -> Real-Imag to Complex/2

== system powerlib_modelsV2/Discrete/Excitation_System/Damping kf.s / (tf.s +1) ==
  In : Inport  Orientation=left  Port=1  LatchInput=off
  1st-Order Discrete Filter : powerlib_extras/Discrete  Control Blocks/Discrete 1st-Order Discrete Filter  Orientation=left  FilterType=Highpass  Tc=tf  Ts=Ts  Initialize=on  Vac_Init=[0 0 60]  Vdc_Init=kf*v0(2)/tf  PlotResponse=off  param1=[1 500 0.1]
  Gain : Gain  Orientation=left  Gain=kf/tf  SaturateOnIntegerOverflow=on
  Out : Outport  Orientation=left
  wires:
  1st-Order Discrete Filter/1 -> Out/1
  Gain/1 -> 1st-Order Discrete Filter/1
  In/1 -> Gain/1

== system powerlib_modelsV2/Discrete/Excitation_System/Exciter  1 / (te.s + ke) ==
  In : Inport  Port=1  LatchInput=off
  1st order Lowpass : powerlib_extras/Discrete  Control Blocks/Discrete 1st-Order Discrete Filter  FilterType=Lowpass  Tc=te/ke  Ts=Ts  Initialize=on  Vac_Init=[0.0 0 60]  Vdc_Init=v0(2)  PlotResponse=off  param1=[1 500 0.1]
  Gain : Gain  Gain=1/ke  SaturateOnIntegerOverflow=on
  Out : Outport
  wires:
  Gain/1 -> 1st order Lowpass/1
  In/1 -> Gain/1
  1st order Lowpass/1 -> Out/1

== system powerlib_modelsV2/Discrete/Excitation_System/Main Regulator ka / (ta.s +1) ==
  In : Inport  Port=1  LatchInput=off
  1st order Lowpass : powerlib_extras/Discrete  Control Blocks/Discrete 1st-Order Discrete Filter  FilterType=Lowpass  Tc=ta  Ts=Ts  Initialize=on  Vac_Init=[0.0 0 60]  Vdc_Init=ke*v0(2)  PlotResponse=off  param1=[1 500 0.1]
  Gain : Gain  Gain=ka  SaturateOnIntegerOverflow=on
  Out : Outport
  wires:
  1st order Lowpass/1 -> Out/1
  In/1 -> Gain/1
  Gain/1 -> 1st order Lowpass/1

== system powerlib_modelsV2/Discrete/Excitation_System/proportionnal saturation ==
  Efd : Inport  Port=1  LatchInput=off
  Vtf : Inport  Port=2  LatchInput=off
  Constant : Constant  Value=kp
  Constant1 : Constant  Value=efmin
  Constant3 : Constant  Value=0
  Data Type  Conversion{,1..3} (4 alike) : DataTypeConversion  SaturateOnIntegerOverflow=on  RndMeth=Zero
  Logical Operator : Logic
  Logical Operator1 : Logic  Operator=NOT  Inputs=1
  Logical Operator2 : Logic  Operator=NOT  Inputs=1
  Product : Product  SaturateOnIntegerOverflow=on  InputSameDT=on
  Product1 : Product  SaturateOnIntegerOverflow=on  InputSameDT=on
  Product2 : Product  SaturateOnIntegerOverflow=on  InputSameDT=on
  Relational Operator : RelationalOperator  Operator===  InputSameDT=on
  Relational Operator1 : RelationalOperator  Operator=<  InputSameDT=on
  Relational Operator2 : RelationalOperator  Operator=>  InputSameDT=on
  Sum : Sum  SaturateOnIntegerOverflow=on  InputSameDT=on
  Sum1 : Sum  Inputs=+++  SaturateOnIntegerOverflow=on  InputSameDT=on
  Vfdmax : Gain  Gain=efmax  SaturateOnIntegerOverflow=on
  Vfdmax1 : Gain  Gain=kp  SaturateOnIntegerOverflow=on
  Ef : Outport  InitialOutput=0
  wires:
  Data Type  Conversion3/1 -> Vfdmax/1
  Relational Operator/1 -> Data Type  Conversion3/1
  Data Type  Conversion2/1 -> Product2/1
  Logical Operator2/1 -> Data Type  Conversion2/1
  Data Type  Conversion1/1 -> Product1/2
  Logical Operator1/1 -> Data Type  Conversion1/1
  Data Type  Conversion/1 -> Product/2
  Logical Operator/1 -> Data Type  Conversion/1
  Product1/1 -> Sum1/2
  Product2/1 -> Sum1/3
  Product/1 -> Sum1/1
  Sum1/1 -> Ef/1
  Efd/1 -> Product/1, Relational Operator1/1, Relational Operator2/1
  Constant1/1 -> Product1/1, Relational Operator2/2
  Relational Operator1/1 -> Logical Operator/2, Logical Operator2/1
  Relational Operator2/1 -> Logical Operator/1, Logical Operator1/1
  Sum/1 -> Relational Operator1/2, Product2/2
  Vfdmax1/1 -> Sum/1
  Vfdmax/1 -> Sum/2
  Constant3/1 -> Relational Operator/2
  Constant/1 -> Relational Operator/1
  Vtf/1 -> Vfdmax1/1

== system powerlib_modelsV2/Discrete/GTO-IGBT Bridge/Diode Logic ==
  note: Note : Block D1 (D2) if D2 (D1) is triggered (no Cs)
  Vak : Inport  Port=1  LatchInput=off
  Ipos : Inport  Port=2  LatchInput=off
  G : Inport  Port=3  LatchInput=off
  0 2 : Constant  Value=0
  0 3 : Constant  Value=Cs==inf
  1 : Logic
  2 : Logic  Operator=OR
  3 : Logic  Operator=OR
  Block D : Selector  Orientation=up  Elements=Selec_Diode  InputPortWidth=nb_switch
  Blocking Diodes : Subsystem
  Data Type  Conversion5 : DataTypeConversion  SaturateOnIntegerOverflow=on  RndMeth=Zero
  Logical Operator3 : Logic  Operator=NOT
  Trig.  Diodes (No Snubber Capacitance) : Subsystem  TreatAsAtomicUnit=on
  b6 : RelationalOperator  Operator=>  InputSameDT=on
  status : Outport  InitialOutput=0
  wires:
  Block D/1 -> 3/2
  3/1 -> Logical Operator3/1
  2/1 -> status/1
  1/1 -> 2/1
  Logical Operator3/1 -> 1/2
  Trig.  Diodes (No Snubber Capacitance)/1(Trig D) -> Block D/1, 2/2
  Blocking Diodes/1(Block.D) -> 3/1
  0 3/1 -> Trig.  Diodes (No Snubber Capacitance)/Enable
  Ipos/1 -> Trig.  Diodes (No Snubber Capacitance)/2(Ipos)
  G/1 -> Trig.  Diodes (No Snubber Capacitance)/1(G), Blocking Diodes/1(G)
  0 2/1 -> b6/2
  Vak/1 -> b6/1
  b6/1 -> Data Type  Conversion5/1
  Data Type  Conversion5/1 -> 1/1

== system powerlib_modelsV2/Discrete/GTO-IGBT Bridge/GTO Logic ==
  Vak : Inport  Port=1  LatchInput=off
  G : Inport  Port=2  LatchInput=off
  " " : RelationalOperator  Operator=>  InputSameDT=on
  "    " : Constant  Value=0
  ". " : Logic
  Data Type  Conversion1 : DataTypeConversion  SaturateOnIntegerOverflow=on  RndMeth=Zero
  Data Type  Conversion2 : DataTypeConversion  SaturateOnIntegerOverflow=on  RndMeth=Zero
  Data Type  Conversion3 : DataTypeConversion  SaturateOnIntegerOverflow=on  RndMeth=Zero
  Vpos : Constant  Value=0
  b : RelationalOperator  Operator=>  InputSameDT=on
  status : Outport  InitialOutput=0
  wires:
  ". "/1 -> status/1
  Vak/1 -> b/1
  Vpos/1 -> b/2
  G/1 -> " "/1
  b/1 -> Data Type  Conversion1/1
  Data Type  Conversion1/1 -> ". "/1
  " "/1 -> Data Type  Conversion2/1
  Data Type  Conversion2/1 -> ". "/2
  "    "/1 -> Data Type  Conversion3/1
  Data Type  Conversion3/1 -> " "/2

== system powerlib_modelsV2/Discrete/GTO-IGBT Bridge/Tail discrete ==
  Iak : Inport  Port=1  LatchInput=off
  switch : Inport  Port=2  LatchInput=off
  Enable : EnablePort  StatesWhenEnabling=reset
  1 : Constant
  Discrete-Time Integrator : DiscreteIntegrator  IntegratorMethod=Integration: Trapezoidal  ExternalReset=falling  SampleTime=Ts  SaturateOnIntegerOverflow=on  ICPrevOutput=DiscIntNeverNeededParam  ICPrevScaledInput=DiscIntNeverNeededParam
  Look-Up Table : Lookup  DialogController=Simulink.DDGSource  InputValues="[  0    Tf+eps Tf+Tt+2*eps  Tf+Tt+3*eps ]"  OutputValues="[  1    0.1*(Tt>0) 0 0]"  SaturateOnIntegerOverflow=on
  Product : Product  SaturateOnIntegerOverflow=on  InputSameDT=on
  Switch : Switch  Threshold=0.5  InputSameDT=on
  Unit Delay3 : UnitDelay  Orientation=left  SampleTime=Ts
  itail : Outport  InitialOutput=0
  wires:
  1/1 -> Discrete-Time Integrator/1
  Discrete-Time Integrator/1 -> Look-Up Table/1
  Look-Up Table/1 -> Product/1
  Product/1 -> itail/1
  Switch/1 -> Unit Delay3/1, Product/2
  Unit Delay3/1 -> Switch/3
  Iak/1 -> Switch/1
  switch/1 -> Discrete-Time Integrator/2, Switch/2

== system powerlib_modelsV2/Discrete/GTO-IGBT Bridge/Vf  ==
  status_GTO : Inport  Port=1  LatchInput=off
  Switch : Switch  Threshold=0.5  InputSameDT=on
  Unit Delay9 : UnitDelay  SampleTime=Ts
  Vf device : Constant  Value=Vf*ones(nb_switch,1)
  Vf diode : Constant  Value=-Vfd*ones(nb_switch,1)
  Vf : Outport  InitialOutput=[0]
  wires:
  Unit Delay9/1 -> Vf/1
  status_GTO/1 -> Switch/2
  Switch/1 -> Unit Delay9/1
  Vf diode/1 -> Switch/3
  Vf device/1 -> Switch/1

== system powerlib_modelsV2/Discrete/HTG/Discrete PID Controller ==
  note: Discrete PID Controller
  note: Pierre Giroux, Gilbert Sybille
      | Power System Simulation Laboratory
      | IREQ, Hydro-Quebc
  Error : Inport  Port=1  LatchInput=off
  "Derivative " : DiscreteTransferFcn  Numerator=[2 -2]  Denominator=[Ts+2*TcD Ts-2*TcD]  SampleTime=Ts
  Discrete-Time Integrator : DiscreteIntegrator  InitialCondition=Init  SampleTime=Ts  SaturateOnIntegerOverflow=on  LimitOutput=on  UpperSaturationLimit=UpperLimit  LowerSaturationLimit=LowerLimit  ICPrevOutput=DiscIntNeverNeededParam  ICPrevScaledInput=DiscIntNeverNeededParam
  Kp4 : Gain  Gain=Kp  SaturateOnIntegerOverflow=on
  Kp5 : Gain  Gain=Ki  SaturateOnIntegerOverflow=on
  Kp6 : Gain  Gain=Kd  SaturateOnIntegerOverflow=on
  Saturation2 : Saturate  UpperLimit=UpperLimit  LowerLimit=LowerLimit
  Sum6 : Sum  Inputs=+++  SaturateOnIntegerOverflow=on  InputSameDT=on
  Out : Outport  InitialOutput=0
  wires:
  Error/1 -> Kp4/1, Kp5/1, Kp6/1
  Sum6/1 -> Saturation2/1
  Kp5/1 -> Discrete-Time Integrator/1
  Kp6/1 -> "Derivative "/1
  Kp4/1 -> Sum6/1
  Discrete-Time Integrator/1 -> Sum6/2
  "Derivative "/1 -> Sum6/3
  Saturation2/1 -> Out/1

== system powerlib_modelsV2/Discrete/HTG/servo-motor ==
  regulator's output : Inport  Port=1  LatchInput=off
  Sum4 : Sum  Inputs=+-  SaturateOnIntegerOverflow=on  InputSameDT=on
  position : DiscreteIntegrator  InitialCondition=go  SampleTime=Ts  SaturateOnIntegerOverflow=on  LimitOutput=on  UpperSaturationLimit=gmax  LowerSaturationLimit=gmin  ICPrevOutput=DiscIntNeverNeededParam  ICPrevScaledInput=DiscIntNeverNeededParam
  servo-motor : Subsystem
  speed limit : Saturate  UpperLimit=vgmax  LowerLimit=vgmin
  gate opening : Outport  InitialOutput=0
  wires:
  position/1 -> Sum4/2, gate opening/1
  speed limit/1 -> position/1
  servo-motor/1(Out) -> speed limit/1
  Sum4/1 -> servo-motor/1(In)
  regulator's output/1 -> Sum4/1

== system powerlib_modelsV2/Discrete/HTG/turbine ==
  dw : Inport  Port=1  LatchInput=off
  gate opening : Inport  Port=2  LatchInput=off
  Constant : Constant  Orientation=left
  Fcn : Fcn  Expr=(u(2)/u(1))^2
  Gain2 : Gain  Orientation=left  Gain=1/tw  SaturateOnIntegerOverflow=on
  Mux : Mux  Inputs=2
  Product : Product  SaturateOnIntegerOverflow=on  InputSameDT=on
  Sum2 : Sum  Inputs=-+  SaturateOnIntegerOverflow=on  InputSameDT=on
  Sum3 : Sum  Orientation=left  Inputs=-+  SaturateOnIntegerOverflow=on  InputSameDT=on
  beta : Gain  Gain=beta  SaturateOnIntegerOverflow=on
  position : DiscreteIntegrator  Orientation=left  InitialCondition=po  SampleTime=Ts  SaturateOnIntegerOverflow=on  UpperSaturationLimit=0  LowerSaturationLimit=0  ICPrevOutput=DiscIntNeverNeededParam  ICPrevScaledInput=DiscIntNeverNeededParam
  turbine gain : Gain  Gain=1/(gmax-gmin)  SaturateOnIntegerOverflow=on
  Pm : Outport  InitialOutput=0
  wires:
  turbine gain/1 -> Mux/1
  gate opening/1 -> turbine gain/1
  Mux/1 -> Fcn/1
  Fcn/1 -> Sum2/2
  Constant/1 -> Sum3/2
  Product/1 -> Pm/1
  Sum3/1 -> Gain2/1
  Gain2/1 -> position/1
  Sum2/1 -> Sum3/1, Product/1
  beta/1 -> Sum2/1
  dw/1 -> beta/1
  position/1 -> Product/2, Mux/2

== system powerlib_modelsV2/Discrete/MBPSS/Discrete Lead-Lag1 ==
  In1 : Inport  Port=1  LatchInput=off
  Discrete State-Space : DiscreteStateSpace  A=Ad  B=Bd  C=Cd  D=Dd  SampleTime=Ts
  Out1 : Outport
  wires:
  Discrete State-Space/1 -> Out1/1
  In1/1 -> Discrete State-Space/1

== system powerlib_modelsV2/Discrete/MBPSS/Discrete Lead-Lag2 ==
  In1 : Inport  Port=1  LatchInput=off
  Discrete State-Space : DiscreteStateSpace  A=Ad  B=Bd  C=Cd  D=Dd  SampleTime=Ts
  Out1 : Outport
  wires:
  In1/1 -> Discrete State-Space/1
  Discrete State-Space/1 -> Out1/1

== system powerlib_modelsV2/Discrete/MBPSS/Discrete Lead-Lag3 ==
  In1 : Inport  Port=1  LatchInput=off
  Discrete State-Space : DiscreteStateSpace  A=Ad  B=Bd  C=Cd  D=Dd  SampleTime=Ts
  Out1 : Outport
  wires:
  In1/1 -> Discrete State-Space/1
  Discrete State-Space/1 -> Out1/1

== system powerlib_modelsV2/Discrete/MBPSS/Discrete Lead-Lag4 ==
  In1 : Inport  Port=1  LatchInput=off
  Discrete State-Space : DiscreteStateSpace  A=Ad  B=Bd  C=Cd  D=Dd  SampleTime=Ts
  Out1 : Outport
  wires:
  Discrete State-Space/1 -> Out1/1
  In1/1 -> Discrete State-Space/1

== system powerlib_modelsV2/Discrete/MBPSS/Discrete Lead-Lag5 ==
  In1 : Inport  Port=1  LatchInput=off
  Discrete State-Space : DiscreteStateSpace  A=Ad  B=Bd  C=Cd  D=Dd  SampleTime=Ts
  Out1 : Outport
  wires:
  Discrete State-Space/1 -> Out1/1
  In1/1 -> Discrete State-Space/1

== system powerlib_modelsV2/Discrete/MBPSS/Discrete Lead-Lag6 ==
  In1 : Inport  Port=1  LatchInput=off
  Discrete State-Space : DiscreteStateSpace  A=Ad  B=Bd  C=Cd  D=Dd  SampleTime=Ts
  Out1 : Outport
  wires:
  In1/1 -> Discrete State-Space/1
  Discrete State-Space/1 -> Out1/1

== system powerlib_modelsV2/Discrete/MBPSS/HF speed sensor ==
  In : Inport  Port=1  LatchInput=off
  Discrete State-Space : DiscreteStateSpace  A=Ad  B=Bd  C=Cd  D=Dd  SampleTime=Ts
  Out : Outport
  wires:
  Discrete State-Space/1 -> Out/1
  In/1 -> Discrete State-Space/1

== system powerlib_modelsV2/Discrete/MBPSS/LF and IF speed sensor ==
  In : Inport  Port=1  LatchInput=off
  Discrete State-Space : DiscreteStateSpace  A=Ad  B=Bd  C=Cd  D=Dd  SampleTime=Ts
  Out : Outport
  wires:
  Discrete State-Space/1 -> Out/1
  In/1 -> Discrete State-Space/1

== system powerlib_modelsV2/Discrete/MBPSS/Transfer function for detailed model (HF) ==
  On : Inport  Port=1  LatchInput=off
  "HFpos " : Inport  Port=2  LatchInput=off
  "HFneg " : Inport  Port=3  LatchInput=off
  Switch1 : Switch  Threshold=0.5  InputSameDT=on
  Switch2 : Switch  Threshold=0.5  InputSameDT=on
  Transfer functions for detailed stabilizer : Subsystem  TreatAsAtomicUnit=on
  Transfer functions for detailed stabilizer1 : Subsystem  TreatAsAtomicUnit=on
  HFpos : Outport
  LFneg : Outport  Port=2
  wires:
  On/1 -> Transfer functions for detailed stabilizer1/Enable, Switch2/2, Switch1/2, Transfer functions for detailed stabilizer/Enable
  Transfer functions for detailed stabilizer1/1(Out1) -> Switch2/1
  Switch2/1 -> LFneg/1
  "HFneg "/1 -> Transfer functions for detailed stabilizer1/1(In1), Switch2/3
  Switch1/1 -> HFpos/1
  "HFpos "/1 -> Switch1/3, Transfer functions for detailed stabilizer/1(In1)
  Transfer functions for detailed stabilizer/1(Out1) -> Switch1/1
